simulink model "untitled"  (Simulink 7.2)
settings: Solver=ode45  StartTime=0.0  StopTime=10.0  RelTol=1e-3
settings Model: Creator=Student  LastModifiedBy=Student

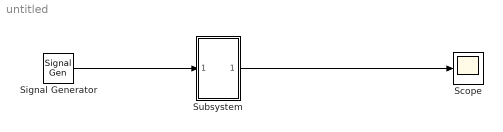
== system untitled ==
  Scope : Scope
  Signal Generator : SignalGenerator
  Subsystem : Subsystem  mask{Ki=1, Kp=0.1, Kd=1}
      mask prompts: Ki "Parametrul Ki"; Kp "Parametrul Kp"; Kd "Parametrul Kd"
  wires:
  Signal Generator/1 -> Subsystem/1(In3)
  Subsystem/1(Out1) -> Scope/1

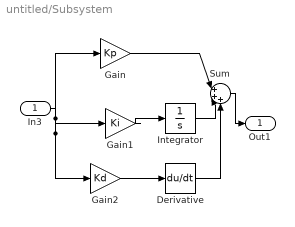
== system untitled/Subsystem ==
  In3 : Inport
  Derivative : Derivative
  Gain : Gain  Gain=Kp  ParameterDataType=sfix(16)  ParameterScaling=2^0  OutDataType=sfix(16)  OutScaling=2^0
  Gain1 : Gain  Gain=Ki  ParameterDataType=sfix(16)  ParameterScaling=2^0  OutDataType=sfix(16)  OutScaling=2^0
  Gain2 : Gain  Gain=Kd  ParameterDataType=sfix(16)  ParameterScaling=2^0  OutDataType=sfix(16)  OutScaling=2^0
  Integrator : Integrator
  Sum : Sum  Inputs=|+++  OutDataType=sfix(16)  OutScaling=2^0
  Out1 : Outport  OutDataType=sfix(16)  OutScaling=2^0
  wires:
  Gain1/1 -> Integrator/1
  Gain2/1 -> Derivative/1
  Gain/1 -> Sum/1
  Integrator/1 -> Sum/2
  Derivative/1 -> Sum/3
  In3/1 -> Gain2/1, Gain1/1, Gain/1
  Sum/1 -> Out1/1
